simulink library "single_phase_pll_sogi"  (R2025b)
settings: Solver=VariableStepAuto  StartTime=0.0  StopTime=10.0  RelTol=1e-3
undefined symbols (not defined in the file): Adrso, Crso, Ldrso, omega_set, ts_inv
settings Model: Creator=dbagn  LastModifiedBy=dbagn

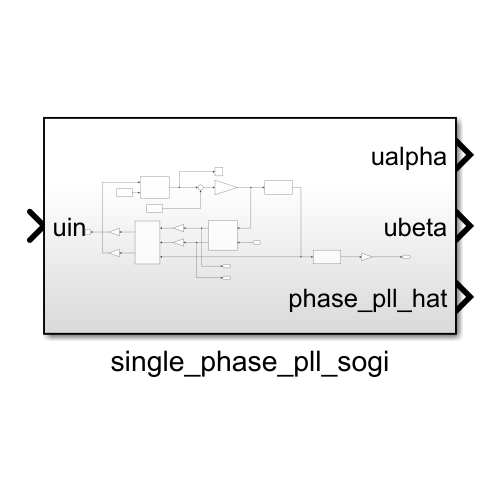
[thumbnail: Simulink's stored preview of the top-level diagram]
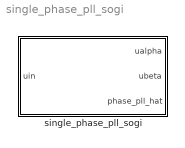
== system single_phase_pll_sogi ==
  single_phase_pll_sogi : Subsystem

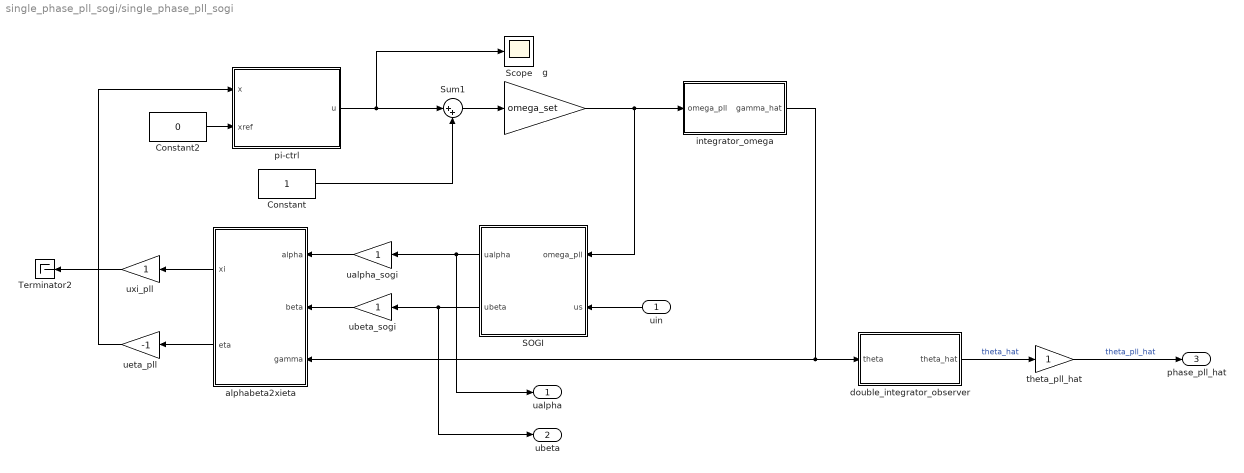
== system single_phase_pll_sogi/single_phase_pll_sogi ==
  uin : Inport
  Constant : Constant
  Constant2 : Constant  Value=0
  SOGI : Subsystem
  Scope : Scope
      settings: ActiveDisplayYMinimum=-0.035554129963767195  ActiveDisplayYMaximum=0.046740470703918784  DataLoggingVariableName=ScopeData16
  Sum1 : Sum  Inputs=|++
  Terminator2 : Terminator
  alphabeta2xieta : MATLAB Function  TreatAsAtomicUnit=on
  double_integrator_observer : Subsystem
  g : Gain  Gain=omega_set
  integrator_omega : Subsystem
  pi-ctrl : Subsystem  mask{kp=1, ki=80, ts=ts_inv, sat_pos=2, sat_neg=-2}
  theta_pll_hat : Gain
  ualpha_sogi : Gain
  ubeta_sogi : Gain
  ueta_pll : Gain  Gain=-1
  uxi_pll : Gain
  ualpha : Outport
  ubeta : Outport  Port=2
  phase_pll_hat : Outport  Port=3
  wires:
  alphabeta2xieta/1(xi) -> uxi_pll/1
  alphabeta2xieta/2(eta) -> ueta_pll/1
  ueta_pll/1 -> pi-ctrl/1(x)
  Sum1/1 -> g/1
  Constant2/1 -> pi-ctrl/2(xref)
  uxi_pll/1 -> Terminator2/1
  SOGI/1(ualpha) -> ualpha/1, ualpha_sogi/1
  SOGI/2(ubeta) -> ubeta/1, ubeta_sogi/1
  integrator_omega/1(gamma_hat) -> alphabeta2xieta/3(gamma), double_integrator_observer/1(theta)
  uin/1 -> SOGI/2(us)
  ualpha_sogi/1 -> alphabeta2xieta/1(alpha)
  ubeta_sogi/1 -> alphabeta2xieta/2(beta)
  Constant/1 -> Sum1/2
  g/1 -> SOGI/1(omega_pll), integrator_omega/1(omega_pll)
  pi-ctrl/1(u) -> Scope/1, Sum1/1
  theta_pll_hat/1 -> phase_pll_hat/1  "theta_pll_hat"
  double_integrator_observer/1(theta_hat) -> theta_pll_hat/1  "theta_hat"

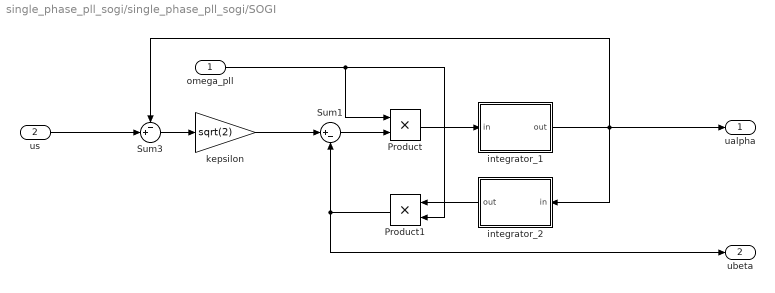
== system single_phase_pll_sogi/single_phase_pll_sogi/SOGI ==
  omega_pll : Inport
  us : Inport  Port=2
  Product : Product
  Product1 : Product
  Sum1 : Sum  Inputs=|+-
  Sum3 : Sum  Inputs=-+|
  integrator_1 : Subsystem
  integrator_2 : Subsystem
  kepsilon : Gain  Gain=sqrt(2)
  ualpha : Outport
  ubeta : Outport  Port=2
  wires:
  us/1 -> Sum3/2
  Sum3/1 -> kepsilon/1
  kepsilon/1 -> Sum1/1
  Sum1/1 -> Product/2
  Product/1 -> integrator_1/1(in)
  integrator_1/1(out) -> Sum3/1, integrator_2/1(in), ualpha/1
  integrator_2/1(out) -> Product1/1
  Product1/1 -> ubeta/1, Sum1/2
  omega_pll/1 -> Product1/2, Product/1

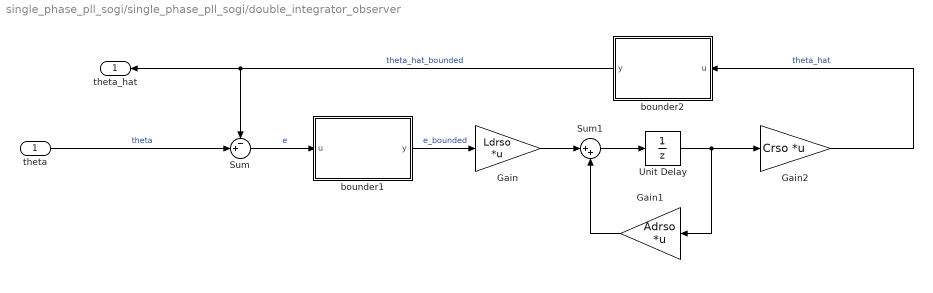
== system single_phase_pll_sogi/single_phase_pll_sogi/double_integrator_observer ==
  theta : Inport
  Gain : Gain  Gain=Ldrso  Multiplication=Matrix(K*u)
  Gain1 : Gain  Gain=Adrso  Multiplication=Matrix(K*u)
  Gain2 : Gain  Gain=Crso  Multiplication=Matrix(K*u)
  Sum : Sum  Inputs=-+|
  Sum1 : Sum  Inputs=|++
  Unit Delay : UnitDelay  SampleTime=-1  HasFrameUpgradeWarning=on
  bounder1 : MATLAB Function  TreatAsAtomicUnit=on
  bounder2 : MATLAB Function  TreatAsAtomicUnit=on
  theta_hat : Outport
  wires:
  Gain/1 -> Sum1/1
  Gain2/1 -> bounder2/1(u)  "theta_hat"
  Gain1/1 -> Sum1/2
  Sum1/1 -> Unit Delay/1
  Sum/1 -> bounder1/1(u)  "e"
  Unit Delay/1 -> Gain1/1, Gain2/1
  theta/1 -> Sum/2  "theta"
  bounder1/1(y) -> Gain/1  "e_bounded"
  bounder2/1(y) -> theta_hat/1, Sum/1  "theta_hat_bounded"

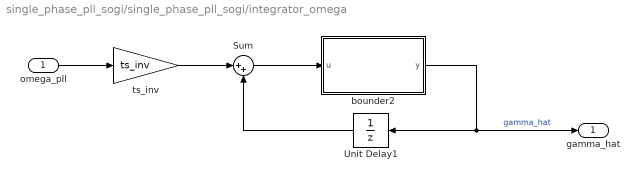
== system single_phase_pll_sogi/single_phase_pll_sogi/integrator_omega ==
  omega_pll : Inport
  Sum : Sum  Inputs=|++
  Unit Delay1 : UnitDelay  SampleTime=-1  HasFrameUpgradeWarning=on
  bounder2 : MATLAB Function  TreatAsAtomicUnit=on
  ts_inv : Gain  Gain=ts_inv
  gamma_hat : Outport
  wires:
  Unit Delay1/1 -> Sum/2
  omega_pll/1 -> ts_inv/1
  Sum/1 -> bounder2/1(u)
  ts_inv/1 -> Sum/1
  bounder2/1(y) -> Unit Delay1/1, gamma_hat/1  "gamma_hat"

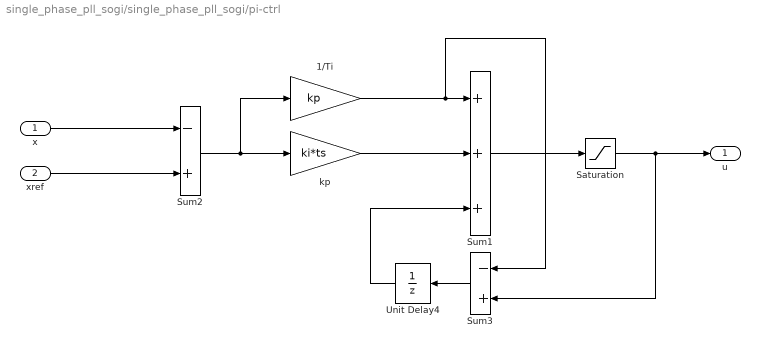
== system single_phase_pll_sogi/single_phase_pll_sogi/pi-ctrl ==
  x : Inport
  xref : Inport  Port=2
  1/Ti : Gain  Gain=kp  SaturateOnIntegerOverflow=on  OutDataTypeStr=Inherit: Same as input  ParamDataTypeStr=Inherit: Same as input
  Saturation : Saturate  UpperLimit=sat_pos  LowerLimit=sat_neg
  Sum1 : Sum  Inputs=+++  SaturateOnIntegerOverflow=on
  Sum2 : Sum  Inputs=-+  SaturateOnIntegerOverflow=on
  Sum3 : Sum  Inputs=-+  SaturateOnIntegerOverflow=on
  Unit Delay4 : UnitDelay  SampleTime=-1  HasFrameUpgradeWarning=on
  kp : Gain  Gain=ki*ts  SaturateOnIntegerOverflow=on  OutDataTypeStr=Inherit: Same as input  ParamDataTypeStr=Inherit: Same as input
  u : Outport
  wires:
  Saturation/1 -> Sum3/2, u/1
  Unit Delay4/1 -> Sum1/3
  Sum1/1 -> Saturation/1
  Sum3/1 -> Unit Delay4/1
  1/Ti/1 -> Sum3/1, Sum1/1
  Sum2/1 -> 1/Ti/1, kp/1
  kp/1 -> Sum1/2
  x/1 -> Sum2/1
  xref/1 -> Sum2/2

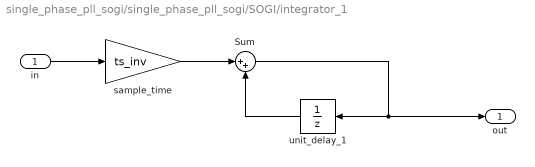
== system single_phase_pll_sogi/single_phase_pll_sogi/SOGI/integrator_1 ==
  in : Inport
  Sum : Sum  Inputs=|++
  sample_time : Gain  Gain=ts_inv
  unit_delay_1 : UnitDelay  SampleTime=-1  HasFrameUpgradeWarning=on
  out : Outport
  wires:
  unit_delay_1/1 -> Sum/2
  in/1 -> sample_time/1
  sample_time/1 -> Sum/1
  Sum/1 -> unit_delay_1/1, out/1

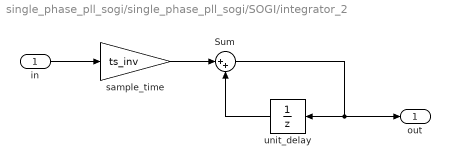
== system single_phase_pll_sogi/single_phase_pll_sogi/SOGI/integrator_2 ==
  in : Inport
  Sum : Sum  Inputs=|++
  sample_time : Gain  Gain=ts_inv
  unit_delay : UnitDelay  SampleTime=-1  HasFrameUpgradeWarning=on
  out : Outport
  wires:
  sample_time/1 -> Sum/1
  Sum/1 -> unit_delay/1, out/1
  in/1 -> sample_time/1
  unit_delay/1 -> Sum/2

== matlab function single_phase_pll_sogi/alphabeta2xieta ==
  data: alpha input; xi output; beta input; gamma input; eta output
function [xi,eta] = alphabeta2xieta(alpha,beta,gamma)
    xi  =  alpha*cos(gamma) + beta*sin(gamma);
    eta = -alpha*sin(gamma) + beta*cos(gamma);
end

== matlab function single_phase_pll_sogi/integrator_omega/bounder2 ==
  data: u input; y output
function y = bounder(u)
    
    y = -pi + mod(u+3*pi,2*pi);
   
end

== matlab function single_phase_pll_sogi/double_integrator_observer/bounder1 ==
  data: u input; y output
function y = bounder(u)
    
    y = -pi + mod(u+3*pi,2*pi);
   
end

== matlab function single_phase_pll_sogi/double_integrator_observer/bounder2 ==
  data: u input; y output
function y = bounder(u)
    
    y = -pi + mod(u+3*pi,2*pi);
   
end
